simulink model "aircraft"  (R2018a)
settings: Solver=VariableStepAuto  StartTime=0.0  StopTime=0  RelTol=1e-3
libraries: aerolibatmos2 x1, motorlib x1
settings Model: Creator=mairon  LastModifiedBy=mairon

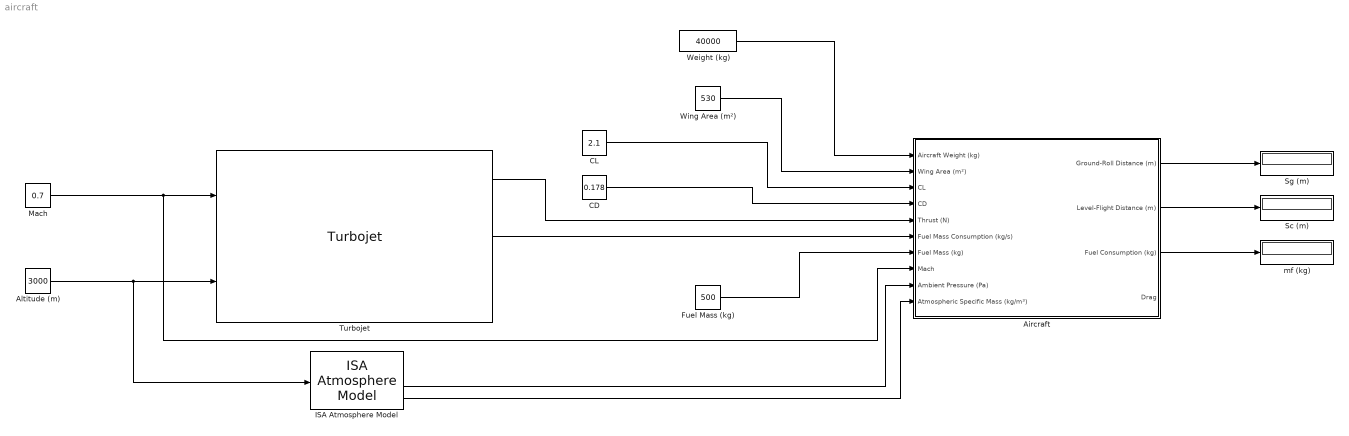
== system aircraft ==
  Aircraft : Subsystem  AncestorBlock=motorlib/Aircraft
  Altitude (m) : Constant  Value=3000
  CD : Constant  Value=0.178
  CL : Constant  Value=2.1
  Fuel Mass (kg) : Constant  Value=500
  ISA Atmosphere Model : aerolibatmos2/ISA Atmosphere Model  custom=off  g=9.80665  gamma=1.4  R=287.0531  L=0.0065  h_trop=11000  h_strat=20000  rho0=1.225  P0=101325  T0=288.15  h0=0
      settings: SourceProductName=Aerospace Blockset
  Mach : Constant  Value=0.7
  Sc (m) : Display
  Sg (m) : Display
  Turbojet : motorlib/Turbojet
      link override Air Flow Mass (kg//s): Value=77
  Weight (kg) : Constant  Value=40000
  Wing Area (m²) : Constant  Value=530
  mf (kg) : Display
  wires:
  Turbojet/1 -> Aircraft/5(Thrust (N))
  Mach/1 -> Aircraft/8(Mach), Turbojet/1
  Altitude (m)/1 -> Turbojet/2, ISA Atmosphere Model/1
  ISA Atmosphere Model/3 -> Aircraft/9(Ambient Pressure (Pa))
  Weight (kg)/1 -> Aircraft/1(Aircraft Weight (kg))
  Wing Area (m²)/1 -> Aircraft/2(Wing Area (m²))
  CD/1 -> Aircraft/4(CD)
  CL/1 -> Aircraft/3(CL)
  Turbojet/2 -> Aircraft/6(Fuel Mass Consumption (kg/s))
  Aircraft/3(Fuel Consumption (kg)) -> mf (kg)/1
  Aircraft/2(Level-Flight Distance (m)) -> Sc (m)/1
  Aircraft/1(Ground-Roll Distance (m)) -> Sg (m)/1
  Fuel Mass (kg)/1 -> Aircraft/7(Fuel Mass (kg))
  ISA Atmosphere Model/4 -> Aircraft/10(Atmospheric Specific Mass (kg/m³))

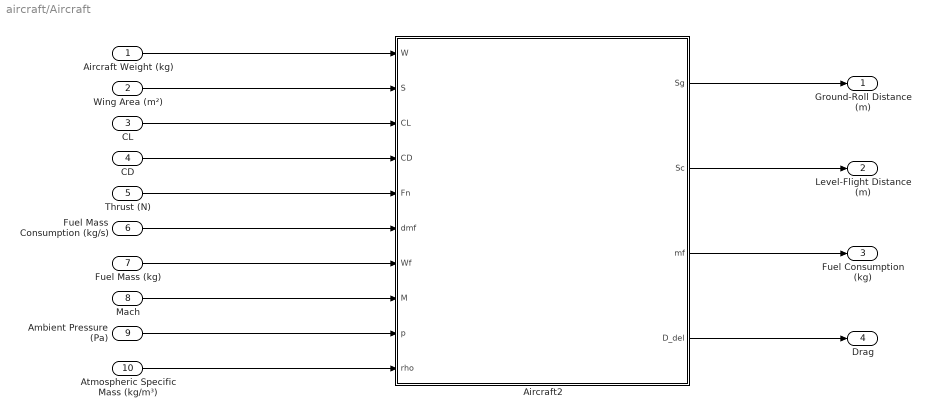
== system aircraft/Aircraft ==
  Aircraft Weight (kg) : Inport
  Wing Area (m²) : Inport  Port=2
  CL : Inport  Port=3
  CD : Inport  Port=4
  Thrust (N) : Inport  Port=5
  Fuel Mass Consumption (kg/s) : Inport  Port=6
  Fuel Mass (kg) : Inport  Port=7
  Mach : Inport  Port=8
  Ambient Pressure (Pa) : Inport  Port=9
  Atmospheric Specific Mass (kg/m³) : Inport  Port=10
  Aircraft2 : MATLAB Function  TreatAsAtomicUnit=on
  Ground-Roll Distance (m) : Outport
  Level-Flight Distance (m) : Outport  Port=2
  Fuel Consumption (kg) : Outport  Port=3
  Drag : Outport  Port=4
  wires:
  Aircraft2/4(D_del) -> Drag/1
  Atmospheric Specific Mass (kg/m³)/1 -> Aircraft2/10(rho)
  Fuel Mass (kg)/1 -> Aircraft2/7(Wf)
  Thrust (N)/1 -> Aircraft2/5(Fn)
  CL/1 -> Aircraft2/3(CL)
  Mach/1 -> Aircraft2/8(M)
  Aircraft2/3(mf) -> Fuel Consumption (kg)/1
  Fuel Mass Consumption (kg/s)/1 -> Aircraft2/6(dmf)
  Ambient Pressure (Pa)/1 -> Aircraft2/9(p)
  Aircraft2/2(Sc) -> Level-Flight Distance (m)/1
  Wing Area (m²)/1 -> Aircraft2/2(S)
  CD/1 -> Aircraft2/4(CD)
  Aircraft Weight (kg)/1 -> Aircraft2/1(W)
  Aircraft2/1(Sg) -> Ground-Roll Distance (m)/1

== matlab function aircraft/Aircraft/Aircraft2 ==
  data: W input; Sg output; S input; CL input; CD input; Fn input; dmf input; Wf input; M input; Sc output; mf output; p input; rho input; D_del output
function [Sg,Sc,mf,D_del] = Aircraft(W,S,CL,CD,Fn,dmf,Wf,M,p,rho)
    g = 9.81;   % [m/s^2]  gravity acceleration
    mu = 0.02;  %          fricction coefficient
    p_std = 101.3e3; % [Pa] standard pressure
    gamma = 1.4;    % specific heat ratio
    
    W = (W+Wf)*g;    % [N] weight
   
    Vstall = sqrt(W/(0.5*CL*rho*S));    % [m/s] stall velocity
    Vlo = Vstall*1.2;                   % [m/s] lift-off velocity
    
    Fn
    a = g*(Fn - mu*W)/W    % [m/s^2] mean acceleration 
    Sg = Vlo^2/(2*a);       % [m] ground-roll distance
    
    dt = Vlo/(2*a)        % [s] ground-roll time
    
    t = Wf/dmf
    Sc = t*(M*340)
    mf=Wf
    
    TSFC = dmf/Fn
    Sc = M*340/g * 1/TSFC * CL/CD * log((W+Wf)/W)
    
    
    % [m] level flight distance
    %Sc = (2/(TSFC*g))*sqrt(2*CL/(S*rho*CD))*(sqrt(W)-sqrt(W-Wf))
    %t = Sc/(M*340)
    
    %mf = dmf*dt
    %mf = dmf*(dt+t)    % [kg]   fuel mass consumption per flight
   
    del = p/p_std;
    
    % power required
    M = 0:0.02:0.9;
    D_del = gamma*0.5*p_std*CD*M.^2*S;
    
    % power available
    Fn_del = Fn/del;
